simulink model "FORWARD_DYNAMICS_MODEL"  (R2024b)
settings: Solver=VariableStepAuto  StartTime=0.0  StopTime=60  RelTol=1e-3
undefined symbols (not defined in the file or in its folder): A_fwd_aug, B_fwd_aug, C_fwd_aug, D_fwd_aug, q1_fwd, q2_fwd, q3_fwd, q4_fwd, q5_fwd, R_fwd
settings Model: Creator=hazza  LastModifiedBy=hazza

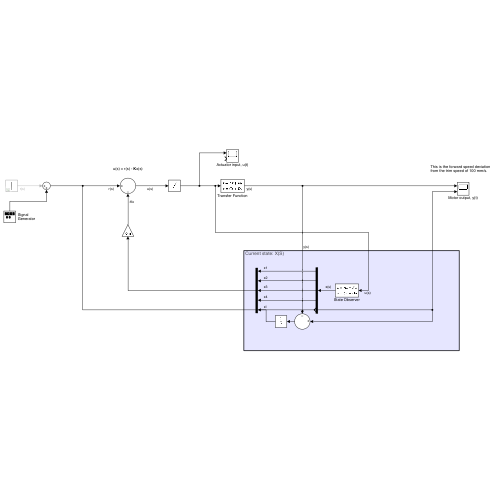
[thumbnail: Simulink's stored preview of the top-level diagram]
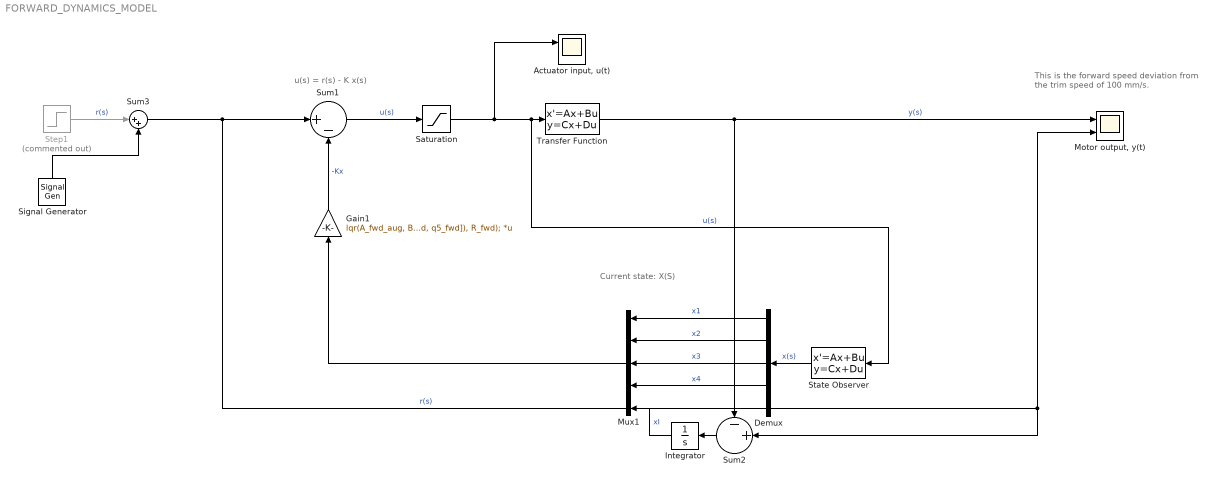
== system FORWARD_DYNAMICS_MODEL ==
  note: This is the forward speed deviation from the trim speed of 100 mm/s.
  note: Current state: X(S)
  note: u(s) = r(s) - K x(s)
  "Actuator input, u(t)" : Scope  NumInputPorts=2
  Demux : Demux  Outputs=5
  Gain1 : Gain  Gain=lqr(A_fwd_aug, B_fwd_aug, diag([q1_fwd, q2_fwd, q3_fwd, q4_fwd, q5_fwd]), R_fwd);  Multiplication=Matrix(K*u)
  Integrator : Integrator
  "Motor output, y(t)" : Scope  NumInputPorts=2
  Mux1 : Mux  Inputs=5
  Saturation : Saturate  UpperLimit=127  LowerLimit=-23  ZeroCross=off
  Signal Generator : SignalGenerator  Amplitude=-1  Frequency=1/5  Units=rad/sec
  State Observer : StateSpace  A=A_fwd_aug  B=B_fwd_aug  C=eye(5)  D=zeros(5,1)  InitialCondition=[0, 0, 0,0, 0]
  Step1 : Step  Commented=on  Time=10  After=10  SampleTime=10
  Sum1 : Sum  Inputs=|+-
  Sum2 : Sum  Inputs=-+|
  Sum3 : Sum  Inputs=|++
  Transfer Function : StateSpace  A=A_fwd_aug  B=B_fwd_aug  C=C_fwd_aug  D=D_fwd_aug  InitialCondition=[0, 0, 0,0, 0]
  wires:
  Gain1/1 -> Sum1/2  "-Kx"
  Transfer Function/1 -> "Motor output, y(t)"/1, Sum2/1  "y(s)"
  Sum3/1 -> Sum1/1, "Motor output, y(t)"/2, Sum2/2  "r(s)"
  Sum1/1 -> Saturation/1  "u(s)"
  Saturation/1 -> State Observer/1, Transfer Function/1, "Actuator input, u(t)"/1  "u(s)"
  Step1/1 -> Sum3/1  "r(s)"
  Signal Generator/1 -> Sum3/2
  Sum2/1 -> Integrator/1
  Integrator/1 -> Mux1/5  "xI"
  State Observer/1 -> Demux/1  "x(s)"
  Mux1/1 -> Gain1/1
  Demux/1 -> Mux1/1  "x1"
  Demux/2 -> Mux1/2  "x2"
  Demux/3 -> Mux1/3  "x3"
  Demux/4 -> Mux1/4  "x4"
